simulink model "SOCPIControlBenchmarkRealVarL"  (R2019b)
settings: Solver=FixedStepAuto  StartTime=0.0  StopTime=50000  FixedStep=0.01  RelTol=1e-3
values from neighbouring files (symbols this model uses):
  kio = 0.6    [benchmarkPIDStartRealVarL.m]
  kpo = 1    [benchmarkPIDStartRealVarL.m]
  maxKi = 1    [benchmarkPIDStartRealVarL.m]
  maxKp = 1    [benchmarkPIDStartRealVarL.m]
  minKi = 0.01    [benchmarkPIDStartRealVarL.m]
  minKp = 0.01    [benchmarkPIDStartRealVarL.m]
  N = 100    [benchmarkPIDStartRealVarL.m]
  optimPeriod = 300    [benchmarkPIDStartRealVarL.m]
  OVLim = 2    [benchmarkPIDStartRealVarL.m]
  refAmplitude = 50    [benchmarkPIDStartRealVarL.m]
  refSignalPeriod = optimPeriod    (= 300)    [benchmarkPIDStartRealVarL.m]
  resetThreshold = 0.1    [benchmarkPIDStartRealVarL.m]
undefined symbols (not defined in the file or in its folder): FORandGCNM, sigbuilder_block
libraries: dspmathops x3, simulink x1
(part 2 of 4)

== matlab function SOCPIControlBenchmarkRealVarL/GCNM/Global NM1 ==
  settings: updateMethod=DISCRETE
  data: f input; y output size=2; kpo input; kio input; OV input; OVLim input; TS input; TSLim input; NM_state_val output; convergenceThresholdBuffer output; NMrestartTolerance input; centroid output; search_on_off input; delay_wait_on_off input; rst input; OVBuffer output; maxLim input; maxLimKi input; minLim input; TSBuffer output; minLimKi input; randKp input; randKi input; YY output
%function [y, NM_state_val,convergenceThresholdBuffer,centroid,BiasRFState1ReflectionCoefficientBuffer]= fcn(f,kpo, kio,BiasRFState1ReflectionCoefficient,BiasRFState1ReflectionCoefficientLim,...
%                                                                                                            NMrestartTolerance, search_on_off, delay_wait_on_off, rst,maxLim,minLim)
function [y, NM_state_val,convergenceThresholdBuffer,centroid,OVBuffer,TSBuffer,YY]= fcn(f,kpo, kio,OV,OVLim,TS,TSLim,...
                                                                                                           NMrestartTolerance, search_on_off, delay_wait_on_off, rst,maxLim,maxLimKi,minLim,minLimKi,randKp,randKi)

% persistent count
persistent NM_state         %Integer definition for states, since enum is not supported
persistent Full_eval_count
persistent usual_delta      %5 percent deltas for non-zero terms
persistent zero_term_delta  %Even smaller delta for zero elements of x
persistent v fv v_r v_e v_m f_r v_c 
persistent yp               %last output when search was on
persistent delay_edge
persistent delay_wait_on_off_z
persistent f_old
persistent windowCounter convergenceThresholdStd gamma1Std gamma2Std delta1Std  ps1Std ps2Std delta2Std
persistent bufferJ bufferGamma1 bufferGamma2 bufferDelta1 bufferDelta2 bufferPS1 bufferPS2;

x=[kpo,kio];  %Initial conditions vector for kp and ki terms

%mead algorithm reset using normal distribution with 1000 choices of initial conditions for Nelder
n = 2;      %Input dimension - needs to be defined as a constant to keep Simulink port width inheretence happy
np1 = n+1;  %Simplex solid dimension
n_r = 1/n;  %Calculate reciprocal at compilation time for mean calculation

%Simplex update coefficients %Can be a function of dimension see Han2010
% alpha = 1;
% beta = 2;
% gamma = 0.5;
% delta = 0.5;

%Adaptive simplex search coefficients: Han2010
alpha = 1;%0.5;
beta = 1 + 2*n_r;%0.5 + 2*n_r;
gamma = 0.75 - 0.5*n_r;
delta = 1 - n_r;

bufferWindow=10;
%NM_state:  
    %0 - Initial   (Initialize vertices)
    %1 - FVE: Full vertex evaluation (with insertion sort after each evaluation)
    %2 - Insertion Sort (After Reflection, Expansion or Contraction Steps)
    %3 - Reflection Entry
    %4 - Reflection Evaluate
    %5 - Expansion
    %6 - Outside Contraction
    %7 - Inside Contraction
    %(8) - Shrink (Implicit on contraction outcome)

%Full_eval_count:
    %Number of initial vertices evaluated
    xin = x(:);         %Force xin to be a column vector
    coder.cinclude('<time.h>')   %% add the library time.c to the generated code
%initialization state of the Nelder Mead
    if isempty(NM_state)
        
        sd=0;
        sd=coder.ceval('time',[]);   %take the seed from the system current time
        rng(sd,'twister');           %initialize the seed of the system using current system seed

        delay_edge = 0;
        yp = xin;
        delay_wait_on_off_z = 0;
        convergenceThresholdStd=100;
        gamma1Std=1;
        gamma2Std=1;
        delta1Std=1;
        delta2Std=1;
        ps1Std=1;
        ps2Std=1;

        windowCounter=1; 
        bufferJ=zeros(1,bufferWindow);
        bufferGamma1=zeros(1,bufferWindow); 
        bufferGamma2=zeros(1,bufferWindow);
        bufferDelta1=zeros(1,bufferWindow); 
        bufferDelta2=zeros(1,bufferWindow); 
        bufferPS1=zeros(1,bufferWindow);
        bufferPS2=zeros(1,bufferWindow);
        
        v = zeros(n,np1);   %Initialize n+1 vertices for simplex
        fv = zeros(1,np1);  %function values at the vertices
        v_m = v(:,1);       %0 vector
        v_r = v_m;          %0 vector    
        v_e = v_m;          %0 vector
        v_c = v_m;          %0 vector
        f_r = 0;          %0 vector

%         usual_delta = 0.01; %original 0.07
        usual_delta = 0.1; %original 0.07
%         zero_term_delta = 0.000025;
        zero_term_delta = 0.0025;
        NM_state = 0;          %Initial state
        Full_eval_count = 1;   %No vertices evaulated, yet

        v(:,1) = xin;
        for j=1:n
            vt = xin;
            if vt(j) ~= 0
                vt(j) = (1 + usual_delta)*vt(j);
            else
                vt(j) = zero_term_delta;
            end
            v(:, j+1) = vt;
        end
        v(2,:)=v(2,:);
    end
    
%restart search when the delay changes    
if (rst==1)  %%Reset the search (Forced reset by external source)
        f_old = 0;
        delay_edge = 0;
        y = xin;
        delay_wait_on_off_z = 0;
        convergenceThresholdStd=0;
       
        windowCounter=1; 
        bufferJ=zeros(1,bufferWindow);
        bufferGamma1=zeros(1,bufferWindow); 
        bufferGamma2=zeros(1,bufferWindow);
        bufferDelta1=zeros(1,bufferWindow); 
        bufferDelta2=zeros(1,bufferWindow); 
        bufferPS1=zeros(1,bufferWindow);
        bufferPS2=zeros(1,bufferWindow);
        
        v = zeros(n,np1);   %Initialize n+1 vertices for simplex
        fv = zeros(1,np1);  %function values at the vertices
        v_m = v(:,1);       %0 vector
        v_r = v_m;          %0 vector    
        v_e = v_m;          %0 vector
        v_c = v_m;          %0 vector
        f_r = 0;          %0 vector

        usual_delta = 0.05;
        zero_term_delta = 0.00025;
        
        
%         usual_delta = 0.1; %Use for force cross decoupling search
%         zero_term_delta = 0.05; %Use for force cross decoupling search

        NM_state = 0;          %Initial state
        Full_eval_count = 1;   %No vertices evaulated, yet

        v(:,1) = [maxLim maxLimKi];
        
        for j=1:n
            vt = [maxLim maxLimKi];
            if vt(j) ~= 0
                vt(j) = (1 + usual_delta)*vt(j);
            else
                vt(j) = zero_term_delta;
            end
            v(:, j+1) = vt;
        end
end



%+++++++++++++ NM search enabling rising flank+++++++++++++++++++++++++++++
% if ((delay_wait_on_off_z == 1) && (delay_wait_on_off == 0))  %falling edge detection for delay_wait_on_off
if ((delay_wait_on_off_z == 0) && (delay_wait_on_off == 1)) %rising edge detection for delay_wait_on_off
    delay_edge = 1;    
    elseif ((delay_wait_on_off_z == 0) && (delay_wait_on_off == 0)) %while level is low
% elseif ((delay_wait_on_off_z == 1) && (delay_wait_on_off == 1)) %while level is high
    delay_edge = 0;
end
    
   
    
%%%++++++++++NM optimization algorithm execution if enable and rising flank are activated   
if ((search_on_off==1) && (delay_edge==1))  




    %restart initialization routine
    gammaCond=(gamma1Std>=OVLim );%|| gamma2Std>=BiasRFState2ReflectionCoefficientLim);
    deltaCond=(gamma2Std>=TSLim);% || delta2Std>=ADVCIPowerSetpointState2Lim);
%     psCond=(ps1Std>=ADVCIPulseQualityDeviationState1Lim || ps2Std>=ADVCIPulseQualityDeviationState2Lim);
    if (abs(convergenceThresholdStd)<= NMrestartTolerance && (gammaCond==1) || deltaCond==1)% || psCond==1) )%&& v_m(1,:)~=0)   %fv(1)>-28       %redo void case, restart the search

           v = zeros(n,np1);   %Initialize n+1 vertices for simplex
           fv = zeros(1,np1);      %function values at the vertices
            v_m = v(:,1);       %0 vector
            v_r = v_m;          %0 vector    
            v_e = v_m;          %0 vector
            v_c = v_m;          %0 vector
            f_r = 0;            %0 vector

%             usual_delta = 0.005;
            usual_delta = 0.1;
            zero_term_delta = 0.025;
            NM_state = 0;          %Initial state
            Full_eval_count = 1;   %No vertices evaulated, yet

            %new initial condition for probabilistic restart
%             v(:,1) = (maxLim*rand(2,1));
            v(1,1) = (maxLim*rand(1,1));
            v(2,1) = (maxLimKi*rand(1,1));
            while ((v(1,1)>maxLim || v(1,1)<minLim) || (v(2,1)>maxLimKi || v(2,1)<minLimKi))==1
                v(:,1) = (maxLim*rand(2,1))+0.01
               
            end



            xin=v(:,1);

            for j=1:n
                vt = xin;
                if vt(j) ~= 0
                    vt(j) = (1 + usual_delta)*vt(j);
                else
                    vt(j) = zero_term_delta;
                end
                v(:, j+1) = vt;
            end   
        convergenceThresholdStd=1;


    end    


    %%%%%%%%%%%%%%%%%%%%%% Nelder Mead State selection  %%%%%%%%%%%%%%%%%%%%%%%     
        switch NM_state  
            case 0 %Vertices has just been initialized
              y = v(:, Full_eval_count); %Write out first vertex for evaluation
              NM_state = 1;

            case 1 %Full vertex evaluation  
                fv(Full_eval_count) = f; %costFunctionJ;  %Read evaluated function value

                j = Full_eval_count;  %New value came in, insert it into sorted list
                while ( (j>1) && (fv(j-1)>fv(j)) ) %Sort ascending
                   temp = fv(j-1);
                   fv(j-1) = fv(j);
                   fv(j) = temp;
                   temp = v(:, j-1);
                   v(:, j-1) = v(:, j); %Also sort corresponding (evaluated) vertices 
                   v(:, j) = temp;
                   j = j-1;
                end

                Full_eval_count = Full_eval_count + 1;            
                if (Full_eval_count <= (np1))
                    y = v(:, Full_eval_count);                
                else
                    Full_eval_count = Full_eval_count - 1; 
                    %NM_state = 3;   %Full vertex evaluation complete -> Reflection 
                    v_sum = xin*0;  %Initialize sum for mean calculation

                    for i=1:n
                        v_sum = v_sum + v(:, i);
                    end

                    v_m = v_sum*n_r; %Centroid
                    v_r  = v_m*(1+alpha) - alpha*v(:, end);
                    y  = v_r;
                    NM_state = 4;   %Reflection Evaluate
                end

            case 2 %Insertion Sort                        
                    j = Full_eval_count;  %New value came in, insert it into list
                       while ( (j>1) && (fv(j-1)>fv(j)) ) %Sort ascending
                           temp = fv(j-1);
                           fv(j-1) = fv(j);
                           fv(j) = temp;
                           temp = v(:, j-1);
                           v(:, j-1) = v(:, j); %Also sort corresponding (evaluated) vertices 
                           v(:, j) = temp;
                           j = j-1;
                       end
                       y  = v_r;
                    NM_state = 3;   %Reflection 

            case 3 %Reflection Entry
                    v_sum = xin*0;  %Initialize sum for mean calculation

                    for i=1:n
                        v_sum = v_sum + v(:, i);
                    end

                    v_m = v_sum*n_r; %Centroid
                    v_r  = v_m*(1+alpha) - alpha*v(:, np1);
                    y  = v_r;
                    NM_state = 4;   %Reflection Evaluate

            case 4 %Reflection Evaluate
                f_r = f; %costFunctionJ;
                if ( (f_r>fv(:, 1)) && (f_r<fv(:, n)) )
                    v(:, np1) = v_r;
                    fv(np1) = f_r;
                    %NM_state = 2;
                    j = Full_eval_count;  %New value came in, insert it into list
                    while ( (j>1) && (fv(j-1)>fv(j)) ) %Sort ascending
                       temp = fv(j-1);
                       fv(j-1) = fv(j);
                       fv(j) = temp;
                       temp = v(:, j-1);
                       v(:, j-1) = v(:, j); %Also sort corresponding (evaluated) vertices 
                       v(:, j) = temp;
                       j = j-1;
                    end
                    %%NM_state = 3;   %Reflection 

                    v_sum = xin*0;  %Initialize sum for mean calculation

                    for i=1:n
                        v_sum = v_sum + v(:, i);
                    end

                    v_m = v_sum*n_r; %Centroid
                    v_r  = v_m*(1+alpha) - alpha*v(:, np1);
                    y  = v_r;
                    NM_state = 4;    %Reflection Evaluate
                elseif (f_r<fv(:, 1))
                    v_e  = v_m*(1-beta) + beta*v_r; 
                    y  = v_e;
                    NM_state = 5;    %Expansion
                else
                    if ( (f_r>=fv(n)) && (f_r<fv(np1)) ) 
                        v_c  = v_m*(1-gamma) + gamma*v_r; 
                        NM_state = 6; %Outside Contraction
                    elseif (f_r>=fv(np1))  
                        v_c  = v_m*(1+gamma) - gamma*v_r; 
                        NM_state = 7; %Inside Contraction
                    end
                    y = v_c;
                end

            case 5 %Expansion
                f_e = f; %costFunctionJ;
                if (f_e<f_r)
                    v(:, end) = v_e;
                    fv(end) = f_e;
                    %NM_state = 2;
                        j = Full_eval_count;  %New value came in, insert it into list
                       while ( (j>1) && (fv(j-1)>fv(j)) ) %Sort ascending
                           temp = fv(j-1);
                           fv(j-1) = fv(j);
                           fv(j) = temp;
                           temp = v(:, j-1);
                           v(:, j-1) = v(:, j); %Also sort corresponding (evaluated) vertices 
                           v(:, j) = temp;
                           j = j-1;
                       end
                    %%NM_state = 3;   %Reflection 

                    v_sum = xin*0;  %Initialize sum for mean calculation

                    for i=1:n
                        v_sum = v_sum + v(:, i);
                    end

                    v_m = v_sum*n_r; %Centroid
                    v_r  = v_m*(1+alpha) - alpha*v(:, np1);
                    y  = v_r;
                    NM_state = 4;   %Reflection Evaluate
                 else
                    v(:, np1) = v_r;
                    fv(np1) = f_r;
                    %NM_state = 2;
                    j = Full_eval_count;  %New value came in, insert it into list
                   while ( (j>1) && (fv(j-1)>fv(j)) ) %Sort ascending
                       temp = fv(j-1);
                       fv(j-1) = fv(j);
                       fv(j) = temp;
                       temp = v(:, j-1);
                       v(:, j-1) = v(:, j); %Also sort corresponding (evaluated) vertices 
                       v(:, j) = temp;
                       j = j-1;
                   end

                   %%NM_state = 3;   %Reflection 

                    v_sum = xin*0;  %Initialize sum for mean calculation

                    for i=1:n
                        v_sum = v_sum + v(:, i);
                    end

                    v_m = v_sum*n_r; %Centroid
                    v_r  = v_m*(1+alpha) - alpha*v(:, np1);
                    y  = v_r;
                    NM_state = 4;   %Reflection Evaluate
                end

           case 6 %Contraction
               f_c = f;%costFunctionJ;
               if (f_c<f_r)
                   v(:, np1) = v_c;
                   fv(np1) = f_c;
                   %NM_state = 2;
                   j = Full_eval_count;  %New value came in, insert it into list
                   while ( (j>1) && (fv(j-1)>fv(j)) ) %Sort ascending
                       temp = fv(j-1);
                       fv(j-1) = fv(j);
                       fv(j) = temp;
                       temp = v(:, j-1);
                       v(:, j-1) = v(:, j); %Also sort corresponding (evaluated) vertices 
                       v(:, j) = temp;
                       j = j-1;
                   end
                    %%NM_state = 3;   %Reflection 

                    v_sum = xin*0;  %Initialize sum for mean calculation

                    for i=1:n
                        v_sum = v_sum + v(:, i);
                    end

                    v_m = v_sum*n_r; %Centroid
                    v_r  = v_m*(1+alpha) - alpha*v(:, np1);
                    y  = v_r;
                    NM_state = 4;   %Reflection Evaluate
               else
                   for j=2:n+1   %Shrink
                     v(:,j) = v(:,1)*(1-delta) + delta*v(:,j);
                   end
                   y = v(:, 2);   %Start with evaluation
                   Full_eval_count = 2; 
                   NM_state = 1; %Full vertex evaluation after shrink
               end
            case 7
                f_c = f;%costFunctionJ;
                   if (f_c<fv(np1))
                       v(:, np1) = v_c;
                       fv(np1) = f_c;
                       %NM_state = 2;
                        j = Full_eval_count;  %New value came in, insert it into list
                        while ( (j>1) && (fv(j-1)>fv(j)) ) %Sort ascending
                           temp = fv(j-1);
                           fv(j-1) = fv(j);
                           fv(j) = temp;
                           temp = v(:, j-1);
                           v(:, j-1) = v(:, j); %Also sort corresponding (evaluated) vertices 
                           v(:, j) = temp;
                           j = j-1;
                        end
                        NM_state = 3;   %Reflection 

                        v_sum = xin*0;  %Initialize sum for mean calculation

                        for i=1:n
                            v_sum = v_sum + v(:, i);
                        end

                        v_m = v_sum*n_r; %Centroid
                        v_r  = v_m*(1+alpha) - alpha*v(:, np1);
                        y  = v_r;
    %                     NM_state = 4;   %Reflection Evaluate
                   else
                       for j=2:n+1 %Shrink
                         v(:,j) = v(:,1)*(1-delta) + delta*v(:,j);
                       end
                       y = v(:,2);   %Start with evaluation
                       Full_eval_count = 2; 
                       NM_state = 1; %Full vertex evaluation after shrink  
                   end     
            otherwise
            y = v(:,1);
         end %End switch NM_states   

         %restart window implemented inside the GCNM function

        bufferJ(windowCounter)=v_m(1,1);                                    %centroid window instead cost function (working without noise)
        bufferGamma1(windowCounter)=OV;
        bufferGamma2(windowCounter)=TS;
%         bufferDelta1(windowCounter)=BiasRFState1PowerSetpointError;
%         bufferDelta2(windowCounter)=BiasRFState2PowerSetpointError;
%         bufferPS1(windowCounter)=  ADVCIPulseQualityDeviationState1;
%         bufferPS2(windowCounter)=  ADVCIPulseQualityDeviationState2;

    %      bufferJ(windowCounter)=f; %cost function window 
         windowCounter=windowCounter+1;
         if windowCounter>bufferWindow
            convergenceThresholdStd=(std(bufferJ));
            gamma1Std=(mean(bufferGamma1));
            gamma2Std=(mean(bufferGamma2));
            delta1Std=(mean(bufferDelta1));
            delta2Std=(mean(bufferDelta2));
            ps1Std=(mean(bufferPS1));
            ps2Std=(mean(bufferPS2));

            windowCounter=1;

         end


    else            %this condition appears when the controller is disabled
         y = yp;
         gammaCond=true;
         deltaCond=true;
%          psCond=true;
     
end

%outputs definitions
     yp = y;
     YY=v;
     NM_state_val = NM_state;
     centroid= v_m; 
     delay_wait_on_off_z = delay_wait_on_off; 
     %sliding window updating
     convergenceThresholdBuffer=convergenceThresholdStd;      %std
     %buffers constraint condition update
             
        OVBuffer=gamma1Std;
        TSBuffer=gamma2Std;
%         BiasRFState1PowerSetpointErrorBuffer=delta1Std;
%         BiasRFState2PowerSetpointErrorBuffer=delta2Std;
%         ADVCIPulseQualityDeviationState1Buffer=ps1Std;
%         ADVCIPulseQualityDeviationState2Buffer=ps2Std;
%      
     
     
end %End of function

== matlab function SOCPIControlBenchmarkRealVarL/GCNM/determinant simplex aware ==
  data: u input; vv1 output; v12 output; v21 output; v1n output; v2n output
function [vv1,v12,v21,v1n,v2n]= fcn(u)
    vv1=u;
    v12=abs(det(vv1(:,2:3)));
    vaux=[vv1(:,1)-vv1(:,2)  vv1(:,1)-vv1(:,3)  ];
    v21=abs(det(vaux));
    
    v1n=norm(vv1(:,2),2);
    v2n=norm(vv1(:,3),2);
    
    
end

== matlab function SOCPIControlBenchmarkRealVarL/GCNM/Cost function2/Cost function ==
  settings: updateMethod=DISCRETE
  data: y input; tsf output; time input; ovf output; epsilon input; r input; period input; yTotal input; samplingTime input; refAmplitude input
function [tsf,ovf] = performance(y,time,epsilon,r,period,yTotal,samplingTime,refAmplitude)
        persistent OV tsFlag yHist counter ts PmAprox;
        
        %initialization state
          if isempty(OV)        
              OV=0;
              PmAprox=0;
              tsFlag=1;
              yHist=zeros(1,round(period/(2*samplingTime)));
%               yHist=zeros(1,round(period/(samplingTime)));
%               ts=0;
              counter=1;
              ts=0*samplingTime;
              tsf=0;
           
          end
          
          yHist(counter)=yTotal;
          
          %overshoot and phase margin calculation 
%           OVCurrent=(max(y)-refAmplitude);
%           tsFlag=max(y);
%           if OVCurrent>OV
%               OV=OVCurrent;
%               ovf=OV;
%               OVPor=abs(OV)/refAmplitude+1e-3;     %overshoot percentage
% %               OVPor=abs(OV-refAmplitude+0.001)/refAmplitude;     %overshoot percentage
%               PmAprox= 100*( -log(OVPor)/ sqrt( pi^2+log(OVPor)^2 )); %approximated phase margin (based on second order system approximation)
%               PmAproxf=PmAprox;
%           else
%               ovf=OV;
%               PmAproxf=PmAprox;
%           end
          
          %calculate settling time each half of the period
          if mod(time,round(period/2))==0    
%           if r==1
            ts=converTimeInvReal(yHist,10,epsilon,refAmplitude);
%             yHist=zeros(1,round(period/2));
            
            tsf=ts*samplingTime;
            counter=0;
            
            OV=(abs(max(yHist)-refAmplitude)/refAmplitude)*100;     %overshoot percentage
            ovf=OV;
          else
              tsf=ts*samplingTime;
              ovf=0;
          end
          
          
          if mod(time,period)==0    %restart constraints after each repetitive period
            OV=0;
            PmAprox=0;
          end
          
          counter=counter+1;
          

end

== matlab function SOCPIControlBenchmarkRealVarL/Original NM1/Cost function/MATLAB Function ==
  settings: updateMethod=DISCRETE
  data: y input; tsf output; time input; ovf output; epsilon input; r input; period input; yTotal input; samplingTime input
function [tsf,ovf] = performance(y,time,epsilon,r,period,yTotal,samplingTime)
        persistent OV tsFlag yHist counter ts;
        
        %initialization state
          if isempty(OV)        
              OV=0;
              tsFlag=1;
              yHist=zeros(1,round(period/(2*samplingTime)));
%               ts=0;
              counter=1;
              ts=0*samplingTime;
              tsf=0;
          end
          
          yHist(counter)=yTotal;
          
          %overshoot calculation
          OVCurrent=max(y);
          if OVCurrent>OV
              OV=OVCurrent;
              ovf=OV;
          else
              ovf=OV;
          end
          
          %calculate settling time each half of the period
          if mod(time,round(period/2))==0    
            ts=converTimeInv1s(yHist,10,epsilon);
%             yHist=zeros(1,round(period/2));
            counter=0;
            tsf=ts*samplingTime;
          else
              tsf=ts*samplingTime;
          end
          
          
          if mod(time,period)==0    %restart constraints after each repetitive period
            OV=0;
          end
          
          counter=counter+1;
          

end

== matlab function SOCPIControlBenchmarkRealVarL/Original NM1/Cost function1/MATLAB Function ==
  settings: updateMethod=DISCRETE
  data: y input; tsf output; time input; ovf output; epsilon input; r input; period input; yTotal input; samplingTime input
function [tsf,ovf] = performance(y,time,epsilon,r,period,yTotal,samplingTime)
        persistent OV tsFlag yHist counter ts;
        
        %initialization state
          if isempty(OV)        
              OV=0;
              tsFlag=1;
              yHist=zeros(1,round(period/(2*samplingTime)));
%               ts=0;
              counter=1;
              ts=0*samplingTime;
              tsf=0;
          end
          
          yHist(counter)=yTotal;
          
          %overshoot calculation
          OVCurrent=max(y);
          if OVCurrent>OV
              OV=OVCurrent;
              ovf=OV;
          else
              ovf=OV;
          end
          
          %calculate settling time each half of the period
          if mod(time,round(period/2))==0    
            ts=converTimeInv1s(yHist,10,epsilon);
%             yHist=zeros(1,round(period/2));
            counter=0;
            tsf=ts*samplingTime;
          else
              tsf=ts*samplingTime;
          end
          
          
          if mod(time,period)==0    %restart constraints after each repetitive period
            OV=0;
          end
          
          counter=counter+1;
          
%           
%           if std(y)<epsilon && tsFlag==1 && r==1 %settling time on the low state
%               ts=time;
%               tsFlag=0;
%           else
%               ts=5;
%           end
          

end
